simulink model "delay_track_sim"  (R2019a)
settings: Solver=VariableStepAuto  StartTime=0.0  StopTime=400000 / (fs_ghz * 1e9)  RelTol=1e-3
undefined symbols (not defined in the file or in its folder): fdesignblkfcn, fs_ghz, gcbh
libraries: dspxfrm3 x2, simulink x2
(part 1 of 7)
settings Model: Creator=jackh  LastModifiedBy=jackh

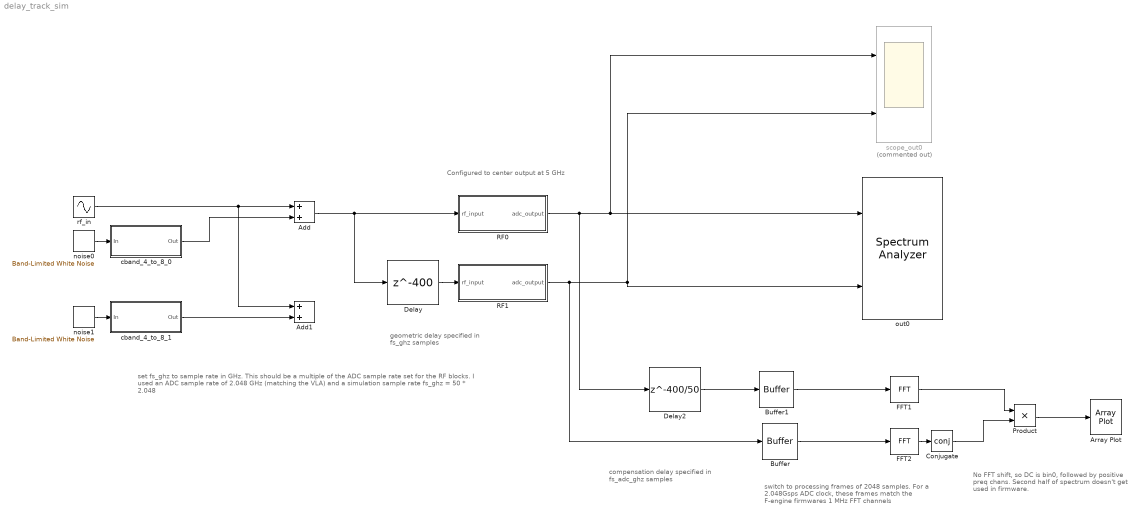
== system delay_track_sim ==
  note: No FFT shift, so DC is bin0, followed
      | by positive preq chans. Second half of spectrum
      | doesn't get used in firmware.
  note: Configured to center output at 5 GHz
  note: compensation delay specified in
      | fs_adc_ghz samples
  note: geometric delay specified
      | in fs_ghz samples
  note: switch to processing frames of 2048 samples.
      | For a 2.048Gsps ADC clock, these frames
      | match the F-engine firmwares 1 MHz FFT channels
  note: set fs_ghz to sample rate in GHz. This should be
      | a multiple of the ADC sample rate set for the
      | RF blocks. I used an ADC sample rate of 2.048 GHz (matching the VLA)
      | and a simulation sample rate fs_ghz = 50 * 2.048
  Add : Sum
  Add1 : Sum
  Array Plot : ArrayPlot
  Buffer : Buffer  N=2048  OutputFrames=off
  Buffer1 : Buffer  N=2048  OutputFrames=off
  Conjugate : Math  Operator=conj  RndMeth=Zero  SaturateOnIntegerOverflow=on
  Delay : Delay  DelayLength=400  InitialCondition=0
  Delay2 : Delay  DelayLength=400/50  InitialCondition=0
  FFT1 : dspxfrm3/FFT  FFTImplementation=Auto  CompMethod=Table lookup  TableOpt=NEW  TableOptActive=Speed  BitRevOrder=off  Normalize=on  InheritFFTLength=on  FFTLength=1024  WrapInput=off  roundingMode=Floor  overflowMode=off  firstCoeffDataTypeStr=Inherit: Same word length as input  firstCoeffLastDataTypeStr=Inherit: Same word length as input  outputMin=[]  outputMax=[]
  FFT2 : dspxfrm3/FFT  FFTImplementation=Auto  CompMethod=Table lookup  TableOpt=NEW  TableOptActive=Speed  BitRevOrder=off  Normalize=on  InheritFFTLength=on  FFTLength=1024  WrapInput=off  roundingMode=Floor  overflowMode=off  firstCoeffDataTypeStr=Inherit: Same word length as input  firstCoeffLastDataTypeStr=Inherit: Same word length as input  outputMin=[]  outputMax=[]
  Product : Product
  RF0 : Subsystem  mask{fshift_hz=0, lo1_ghz=16, lo2_ghz=13.5, adc_fs_ghz=2.048}
      mask prompts: fshift_hz "Fshift in Hz"; lo1_ghz "LO1 frequency in GHz"; lo2_ghz "LO2 frequency in GHz"; adc_fs_ghz "Output sample rate in GHz"
  RF1 : Subsystem  mask{fshift_hz=0, lo1_ghz=16, lo2_ghz=13.5, adc_fs_ghz=2.048}
      mask prompts: fshift_hz "Fshift in Hz"; lo1_ghz "LO1 frequency in GHz"; lo2_ghz "LO2 frequency in GHz"; adc_fs_ghz "Output sample rate in GHz"
  cband_4_to_8_0 : Subsystem  DialogController=fdesignblkfcn  InitFcn=fdesignblkfcn(gcbh, {'InitFcn'});  mask(Bandpass Filter){}
      mask help: Design a bandpass filter
      settings: CopyFcn=fdesignblkfcn(gcbh, {'CopyFcn'});
      mask Help: helpview(mapfilelocation('dsp'), 'dspbandpassfilter');
      mask Display: disp('Bandpass');
  cband_4_to_8_1 : Subsystem  DialogController=fdesignblkfcn  InitFcn=fdesignblkfcn(gcbh, {'InitFcn'});  mask(Bandpass Filter){}
      mask help: Design a bandpass filter
      settings: CopyFcn=fdesignblkfcn(gcbh, {'CopyFcn'});
      mask Help: helpview(mapfilelocation('dsp'), 'dspbandpassfilter');
      mask Display: disp('Bandpass');
  noise0 : simulink/Sources/Band-Limited White Noise  Cov=[1e-8]  Ts=1/(fs_ghz*1e9)  seed=[23341]
  noise1 : simulink/Sources/Band-Limited White Noise  Cov=[1e-8]  Ts=1/(fs_ghz*1e9)  seed=[12345]
  out0 : SpectrumAnalyzer  NumInputPorts=2
  rf_in : Sin  Amplitude=100  Frequency=4.75e9 * 2 * pi  SampleTime=1/(fs_ghz*1e9)
  scope_out0 : Scope  Commented=on  NumInputPorts=2
  wires:
  cband_4_to_8_0/1(Out) -> Add/2
  Add/1 -> Delay/1, RF0/1(rf_input)
  cband_4_to_8_1/1(Out) -> Add1/2
  FFT1/1 -> Product/1
  FFT2/1 -> Conjugate/1
  Conjugate/1 -> Product/2
  Product/1 -> Array Plot/1
  RF0/1(adc_output) -> Delay2/1, out0/1, scope_out0/1
  noise0/1 -> cband_4_to_8_0/1(In)
  noise1/1 -> cband_4_to_8_1/1(In)
  rf_in/1 -> Add/1, Add1/1
  Buffer/1 -> FFT2/1
  Buffer1/1 -> FFT1/1
  Delay/1 -> RF1/1(rf_input)
  RF1/1(adc_output) -> Buffer/1, scope_out0/2, out0/2
  Delay2/1 -> Buffer1/1

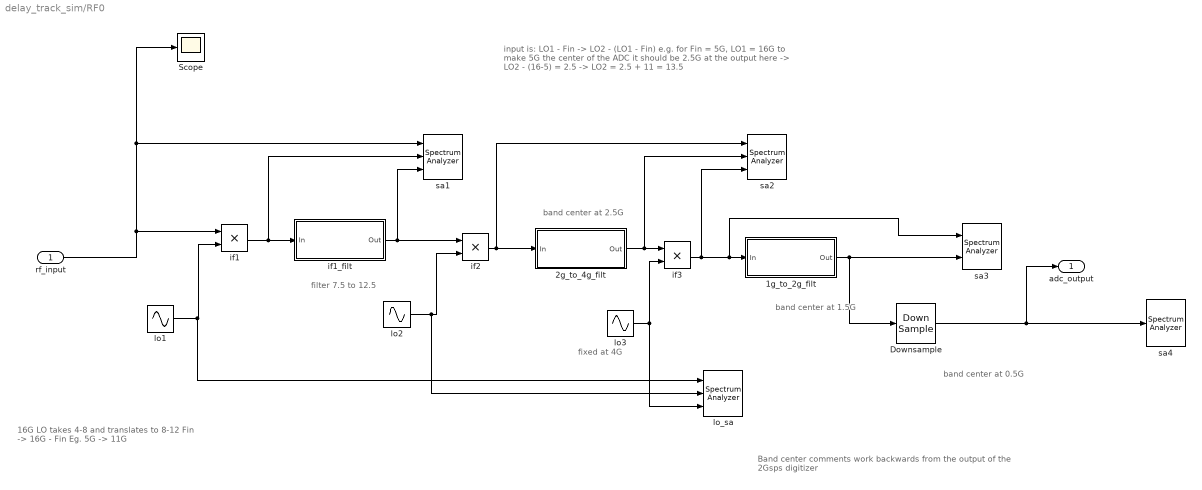
== system delay_track_sim/RF0 ==
  note: input is:
      | LO1 - Fin -> LO2 - (LO1 - Fin)
      | e.g.
      | for Fin = 5G, LO1 = 16G
      | to make 5G the center of the ADC it should be 2.5G at the output here
      | -> LO2 - (16-5) = 2.5
      | -> LO2 = 2.5 + 11 = 13.5
  note: Band center comments work backwards
      | from the output of the 2Gsps digitizer
  note: fixed at 4G
  note: band center at 1.5G
  note: band center at 0.5G
  note: filter 7.5 to 12.5
  note: 16G LO takes 4-8 and translates to 8-12
      |
      | Fin -> 16G - Fin
      |
      | Eg. 5G -> 11G
  note: band center at 2.5G
  rf_input : Inport
  1g_to_2g_filt : Subsystem  DialogController=fdesignblkfcn  InitFcn=fdesignblkfcn(gcbh, {'InitFcn'});  mask(Bandpass Filter){}
      mask help: Design a bandpass filter
      settings: CopyFcn=fdesignblkfcn(gcbh, {'CopyFcn'});
      mask Help: helpview(mapfilelocation('dsp'), 'dspbandpassfilter');
      mask Display: disp('Bandpass');
  2g_to_4g_filt : Subsystem  DialogController=fdesignblkfcn  InitFcn=fdesignblkfcn(gcbh, {'InitFcn'});  mask(Bandpass Filter){}
      mask help: Design a bandpass filter
      settings: CopyFcn=fdesignblkfcn(gcbh, {'CopyFcn'});
      mask Help: helpview(mapfilelocation('dsp'), 'dspbandpassfilter');
      mask Display: disp('Bandpass');
  Downsample : DownSample  N=fs_ghz/adc_fs_ghz  RateOptions=Allow multirate processing
  Scope : Scope
  if1 : Product
  if1_filt : Subsystem  DialogController=fdesignblkfcn  InitFcn=fdesignblkfcn(gcbh, {'InitFcn'});  mask(Bandpass Filter){}
      mask help: Design a bandpass filter
      settings: CopyFcn=fdesignblkfcn(gcbh, {'CopyFcn'});
      mask Help: helpview(mapfilelocation('dsp'), 'dspbandpassfilter');
      mask Display: disp('Bandpass');
  if2 : Product
  if3 : Product
  lo1 : Sin  Frequency=lo1_ghz * 1e9 * 2 * pi  SampleTime=1/(fs_ghz * 1e9)
  lo2 : Sin  Frequency=(lo2_ghz*1e9 + fshift_hz) * 2 * pi  SampleTime=1/(fs_ghz*1e9)
  lo3 : Sin  Frequency=4e9 * 2 * pi  SampleTime=1/(fs_ghz * 1e9)
  lo_sa : SpectrumAnalyzer  NumInputPorts=3
  sa1 : SpectrumAnalyzer  NumInputPorts=3
  sa2 : SpectrumAnalyzer  NumInputPorts=3
  sa3 : SpectrumAnalyzer  NumInputPorts=2
  sa4 : SpectrumAnalyzer
  adc_output : Outport
  wires:
  Downsample/1 -> adc_output/1, sa4/1
  if2/1 -> 2g_to_4g_filt/1(In), sa2/1
  2g_to_4g_filt/1(Out) -> if3/1, sa2/2
  rf_input/1 -> sa1/1, Scope/1, if1/1
  if3/1 -> sa3/1, 1g_to_2g_filt/1(In), sa2/3
  if1/1 -> sa1/2, if1_filt/1(In)
  if1_filt/1(Out) -> sa1/3, if2/1
  1g_to_2g_filt/1(Out) -> Downsample/1, sa3/2
  lo1/1 -> lo_sa/1, if1/2
  lo2/1 -> lo_sa/2, if2/2
  lo3/1 -> lo_sa/3, if3/2

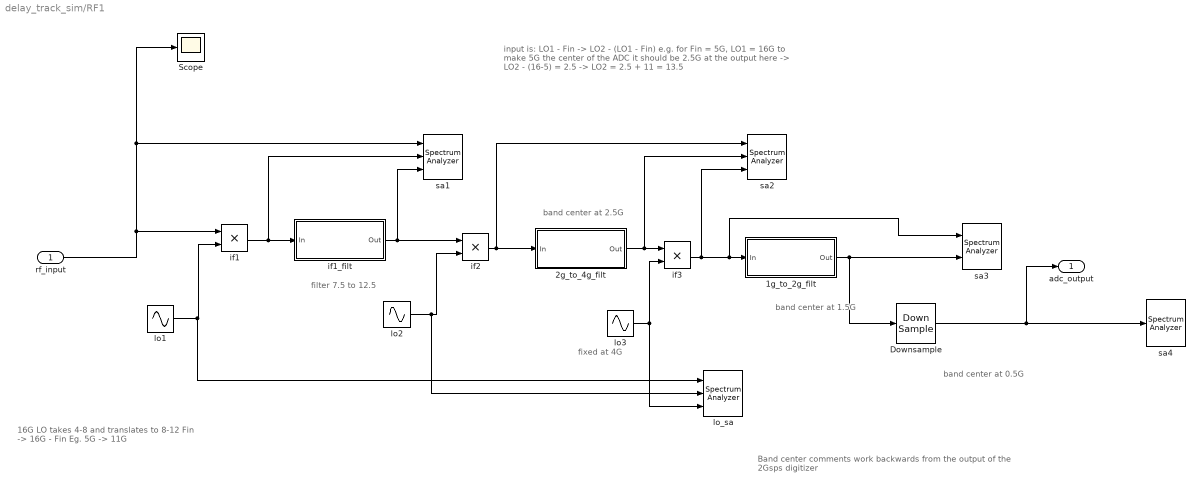
== system delay_track_sim/RF1 ==
  note: band center at 2.5G
  note: 16G LO takes 4-8 and translates to 8-12
      |
      | Fin -> 16G - Fin
      |
      | Eg. 5G -> 11G
  note: filter 7.5 to 12.5
  note: band center at 0.5G
  note: band center at 1.5G
  note: fixed at 4G
  note: Band center comments work backwards
      | from the output of the 2Gsps digitizer
  note: input is:
      | LO1 - Fin -> LO2 - (LO1 - Fin)
      | e.g.
      | for Fin = 5G, LO1 = 16G
      | to make 5G the center of the ADC it should be 2.5G at the output here
      | -> LO2 - (16-5) = 2.5
      | -> LO2 = 2.5 + 11 = 13.5
  rf_input : Inport
  1g_to_2g_filt : Subsystem  DialogController=fdesignblkfcn  InitFcn=fdesignblkfcn(gcbh, {'InitFcn'});  mask(Bandpass Filter){}
      mask help: Design a bandpass filter
      settings: CopyFcn=fdesignblkfcn(gcbh, {'CopyFcn'});
      mask Help: helpview(mapfilelocation('dsp'), 'dspbandpassfilter');
      mask Display: disp('Bandpass');
  2g_to_4g_filt : Subsystem  DialogController=fdesignblkfcn  InitFcn=fdesignblkfcn(gcbh, {'InitFcn'});  mask(Bandpass Filter){}
      mask help: Design a bandpass filter
      settings: CopyFcn=fdesignblkfcn(gcbh, {'CopyFcn'});
      mask Help: helpview(mapfilelocation('dsp'), 'dspbandpassfilter');
      mask Display: disp('Bandpass');
  Downsample : DownSample  N=fs_ghz/adc_fs_ghz  RateOptions=Allow multirate processing
  Scope : Scope
  if1 : Product
  if1_filt : Subsystem  DialogController=fdesignblkfcn  InitFcn=fdesignblkfcn(gcbh, {'InitFcn'});  mask(Bandpass Filter){}
      mask help: Design a bandpass filter
      settings: CopyFcn=fdesignblkfcn(gcbh, {'CopyFcn'});
      mask Help: helpview(mapfilelocation('dsp'), 'dspbandpassfilter');
      mask Display: disp('Bandpass');
  if2 : Product
  if3 : Product
  lo1 : Sin  Frequency=lo1_ghz * 1e9 * 2 * pi  SampleTime=1/(fs_ghz * 1e9)
  lo2 : Sin  Frequency=(lo2_ghz*1e9 + fshift_hz) * 2 * pi  SampleTime=1/(fs_ghz*1e9)
  lo3 : Sin  Frequency=4e9 * 2 * pi  SampleTime=1/(fs_ghz * 1e9)
  lo_sa : SpectrumAnalyzer  NumInputPorts=3
  sa1 : SpectrumAnalyzer  NumInputPorts=3
  sa2 : SpectrumAnalyzer  NumInputPorts=3
  sa3 : SpectrumAnalyzer  NumInputPorts=2
  sa4 : SpectrumAnalyzer
  adc_output : Outport
  wires:
  lo3/1 -> if3/2, lo_sa/3
  lo2/1 -> if2/2, lo_sa/2
  lo1/1 -> if1/2, lo_sa/1
  1g_to_2g_filt/1(Out) -> sa3/2, Downsample/1
  if1_filt/1(Out) -> if2/1, sa1/3
  if1/1 -> if1_filt/1(In), sa1/2
  if3/1 -> sa2/3, 1g_to_2g_filt/1(In), sa3/1
  rf_input/1 -> if1/1, Scope/1, sa1/1
  2g_to_4g_filt/1(Out) -> sa2/2, if3/1
  if2/1 -> sa2/1, 2g_to_4g_filt/1(In)
  Downsample/1 -> sa4/1, adc_output/1

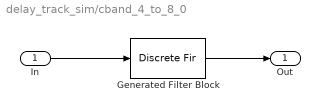
== system delay_track_sim/cband_4_to_8_0 ==
  In : Inport
  Generated Filter Block : DiscreteFir  Tag=BlockMethodSubSystem  Coefficients=[-9.40094334225731145e-05 -6.57335329822327186e-05 1.32894792001724368e-05 0.000134559058517748424 0.000277936305882253612 0.000414699232132098247 0.000512636064975988365 0.000542480818344473047 0.000484608636541211375 0.000334635227065140138 0.000106521266150224518 -0.00016793806988651982 -0.000443730870127158567 -0.000670944573551014874 -0.000805375180787633121 -0.000819188075913799977 -0.000708981167312832013 -0.000498824743569846246 -0.000236769281391713434 1.5203544332798152e-05 0.000196071777662499826 0.000262234950789153 0.00020136374340029727 3.95409230838828136e-05 -0.000161189091747555358 -0.000315568714700558729 -0.000336199033950288569 -0.000158434546317144811 0.000237060749983095386 0.000810486359802426045 0.00146274357449518544 0.00205091179934143017 0.00241746714197546954 0.00242749537258047125 0.00200534282778644293 0.00116125186658666644 -3.15157742191004583e-18 -0.00129271620505455294 -0.00248516845896724512 -0.00334921577167213895 -0.00371366539057864592 -0.00350831585599136993 -0.00278671416575157612 -0.00171994678369694239 -0.00056047250948902574 0.000417403157207240716 0.000987193246086869557 0.00103297042357498327 0.000588304387599879598 -0.000160939057919878934 -0.000914126130308830697 -0.00132790755313672969 -0.00110754221024641879 -9.57941142787334198e-05 0.00166381587745433805 0.0039083829069295169 0.00619114734763202747 0.00796797443878280096 0.0087184646970970784 0.00807514580482832263 0.00592966515775395636 0.00248769544754488163 -0.00174568080501794759 -0.00605290349817866509 -0.0096485217876357797 -0.0118514346212249561 -0.0122455147869713152 -0.0107889199476976679 -0.00784163544724328886 -0.0040982275168528438 -0.000434822758380985362 0.0022990180208078189 0.0034968782761721196 0.00296786474365927887 0.0010183703935355325 -0.0015852430988900581 -0.00377519369945273622 -0.00443512989009648556 -0.00269518342804392829 0.00179789767968238103 0.00870320344535378647 0.0169531782155573456 0.0248900360785084297 0.0305583794359089132 0.0321046328349279542 0.0282053415660585664 0.0184329407693223819 0.0034733117399157673 -0.0148656808474887919 -0.0338756640577210708 -0.0503732359862203646 -0.0612589748306400367 -0.0641072262295103168 -0.057671301312918144 -0.0421993420028486943 -0.0194887428317629535 0.00734427980764252447 0.034348129483717689 0.057389809708176677 0.0728614410164006021 0.0783084570220021481 0.0728614410164006021 0.057389809708176677 0.034348129483717689 0.00734427980764252447 -0.0194887428317629535 -0.0421993420028486943 -0.057671301312918144 -0.0641072262295103168 -0.0612589748306400367 -0.0503732359862203646 -0.0338756640577210708 -0.0148656808474887919 0.0034733117399157673 0.0184329407693223819 0.0282053415660585664 0.0321046328349279542 0.0305583794359089132 0.0248900360785084297 0.0169531782155573456 0.00870320344535378647 0.00179789767968238103 -0.00269518342804392829 -0.00443512989009648556 -0.00377519369945273622 -0.0015852430988900581 0.0010183703935355325 0.00296786474365927887 0.0034968782761721196 0.0022990180208078189 -0.000434822758380985362 -0.0040982275168528438 -0.00784163544724328886 -0.0107889199476976679 -0.0122455147869713152 -0.0118514346212249561 -0.0096485217876357797 -0.00605290349817866509 -0.00174568080501794759 0.00248769544754488163 0.00592966515775395636 0.00807514580482832263 0.0087184646970970784 0.00796797443878280096 0.00619114734763202747 0.0039083829069295169 0.00166381587745433805 -9.57941142787334198e-05 -0.00110754221024641879 -0.00132790755313672969 -0.000914126130308830697 -0.000160939057919878934 0.000588304387599879598 0.00103297042357498327 0.000987193246086869557 0.000417403157207240716 -0.00056047250948902574 -0.00171994678369694239 -0.00278671416575157612 -0.00350831585599136993 -0.00371366539057864592 -0.00334921577167213895 -0.00248516845896724512 -0.00129271620505455294 -3.15157742191004583e-18 0.00116125186658666644 0.00200534282778644293 0.00242749537258047125 0.00241746714197546954 0.00205091179934143017 0.00146274357449518544 ...(+728 chars)]  InputProcessing=Columns as channels (frame based)
  Out : Outport
  wires:
  Generated Filter Block/1 -> Out/1
  In/1 -> Generated Filter Block/1

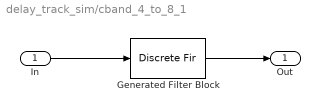
== system delay_track_sim/cband_4_to_8_1 ==
  In : Inport
  Generated Filter Block : DiscreteFir  Tag=BlockMethodSubSystem  Coefficients=[-9.40094334225731145e-05 -6.57335329822327186e-05 1.32894792001724368e-05 0.000134559058517748424 0.000277936305882253612 0.000414699232132098247 0.000512636064975988365 0.000542480818344473047 0.000484608636541211375 0.000334635227065140138 0.000106521266150224518 -0.00016793806988651982 -0.000443730870127158567 -0.000670944573551014874 -0.000805375180787633121 -0.000819188075913799977 -0.000708981167312832013 -0.000498824743569846246 -0.000236769281391713434 1.5203544332798152e-05 0.000196071777662499826 0.000262234950789153 0.00020136374340029727 3.95409230838828136e-05 -0.000161189091747555358 -0.000315568714700558729 -0.000336199033950288569 -0.000158434546317144811 0.000237060749983095386 0.000810486359802426045 0.00146274357449518544 0.00205091179934143017 0.00241746714197546954 0.00242749537258047125 0.00200534282778644293 0.00116125186658666644 -3.15157742191004583e-18 -0.00129271620505455294 -0.00248516845896724512 -0.00334921577167213895 -0.00371366539057864592 -0.00350831585599136993 -0.00278671416575157612 -0.00171994678369694239 -0.00056047250948902574 0.000417403157207240716 0.000987193246086869557 0.00103297042357498327 0.000588304387599879598 -0.000160939057919878934 -0.000914126130308830697 -0.00132790755313672969 -0.00110754221024641879 -9.57941142787334198e-05 0.00166381587745433805 0.0039083829069295169 0.00619114734763202747 0.00796797443878280096 0.0087184646970970784 0.00807514580482832263 0.00592966515775395636 0.00248769544754488163 -0.00174568080501794759 -0.00605290349817866509 -0.0096485217876357797 -0.0118514346212249561 -0.0122455147869713152 -0.0107889199476976679 -0.00784163544724328886 -0.0040982275168528438 -0.000434822758380985362 0.0022990180208078189 0.0034968782761721196 0.00296786474365927887 0.0010183703935355325 -0.0015852430988900581 -0.00377519369945273622 -0.00443512989009648556 -0.00269518342804392829 0.00179789767968238103 0.00870320344535378647 0.0169531782155573456 0.0248900360785084297 0.0305583794359089132 0.0321046328349279542 0.0282053415660585664 0.0184329407693223819 0.0034733117399157673 -0.0148656808474887919 -0.0338756640577210708 -0.0503732359862203646 -0.0612589748306400367 -0.0641072262295103168 -0.057671301312918144 -0.0421993420028486943 -0.0194887428317629535 0.00734427980764252447 0.034348129483717689 0.057389809708176677 0.0728614410164006021 0.0783084570220021481 0.0728614410164006021 0.057389809708176677 0.034348129483717689 0.00734427980764252447 -0.0194887428317629535 -0.0421993420028486943 -0.057671301312918144 -0.0641072262295103168 -0.0612589748306400367 -0.0503732359862203646 -0.0338756640577210708 -0.0148656808474887919 0.0034733117399157673 0.0184329407693223819 0.0282053415660585664 0.0321046328349279542 0.0305583794359089132 0.0248900360785084297 0.0169531782155573456 0.00870320344535378647 0.00179789767968238103 -0.00269518342804392829 -0.00443512989009648556 -0.00377519369945273622 -0.0015852430988900581 0.0010183703935355325 0.00296786474365927887 0.0034968782761721196 0.0022990180208078189 -0.000434822758380985362 -0.0040982275168528438 -0.00784163544724328886 -0.0107889199476976679 -0.0122455147869713152 -0.0118514346212249561 -0.0096485217876357797 -0.00605290349817866509 -0.00174568080501794759 0.00248769544754488163 0.00592966515775395636 0.00807514580482832263 0.0087184646970970784 0.00796797443878280096 0.00619114734763202747 0.0039083829069295169 0.00166381587745433805 -9.57941142787334198e-05 -0.00110754221024641879 -0.00132790755313672969 -0.000914126130308830697 -0.000160939057919878934 0.000588304387599879598 0.00103297042357498327 0.000987193246086869557 0.000417403157207240716 -0.00056047250948902574 -0.00171994678369694239 -0.00278671416575157612 -0.00350831585599136993 -0.00371366539057864592 -0.00334921577167213895 -0.00248516845896724512 -0.00129271620505455294 -3.15157742191004583e-18 0.00116125186658666644 0.00200534282778644293 0.00242749537258047125 0.00241746714197546954 0.00205091179934143017 0.00146274357449518544 ...(+728 chars)]  InputProcessing=Columns as channels (frame based)
  Out : Outport
  wires:
  In/1 -> Generated Filter Block/1
  Generated Filter Block/1 -> Out/1
